simulink model "verify_AIV_WetBulbTemperature_mdl"  (R2016b)
settings: Solver=VariableStepDiscrete  StartTime=0.0  StopTime=10.0  MaxStep=0.1  RelTol=1e-3  EnableMultiTasking=on
undefined symbols (not defined in the file or in its folder): rel_hum2x
libraries: carnot x2
settings Model: Creator=drhf  LastModifiedBy=drhf
settings DataIOCC: LimitDataPoints=on  SaveFormat=Array
settings OptimizationCC: ExpressionDepthLimit=2147483647  LifeSpan=inf
settings DebuggingCC: UnderspecifiedInitializationDetection=Classic  MergeDetectMultiDrivingBlocksExec=none  SolverPrmCheckMsg=warning  StateNameClashWarn=warning  SFUnexpectedBacktrackingDiag=warning  SFNoUnconditionalDefaultTransitionDiag=warning  SFExecutionAtInitializationDiag=none
settings HardwareCC: ProdBitPerPointer=32  ProdBitPerSizeT=32  ProdBitPerPtrDiffT=32  ProdLargestAtomicFloat=None  ProdIntDivRoundTo=Undefined  ProdEndianess=Unspecified  ProdWordSize=32  ProdHWDeviceType=32-bit Generic
settings ModelReferenceCC: PropagateSignalLabelsOutOfModel=off
settings GRTTargetCC: TargetLangStandard=C89/C90 (ANSI)  GeneratePreprocessorConditionals=Disable all  CombineOutputUpdateFcns=off  GRTInterface=on
settings ConfigComp: CovMetricSettings=dw  CovHtmlReporting=on  CovSaveCumulativeToWorkspaceVar=on  CovSaveSingleToWorkspaceVar=on  CovExternalEMLEnable=off

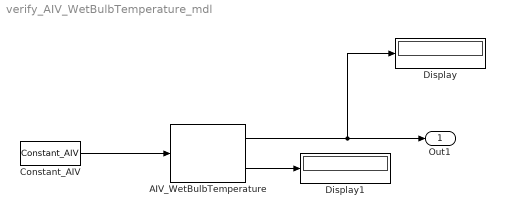
== system verify_AIV_WetBulbTemperature_mdl ==
  AIV_WetBulbTemperature : carnot/Basic/Material_Properties/AIV_WetBulbTemperature
  Constant_AIV : carnot/Source/Ventilation/Constant_AIV  Tsens=20  Tcon=20  Trad=20  mw=rel_hum2x(20,1e5,50)  mco=500/1e6  rhoair=1.2  cpair=1004  pair=100000  nair=0.5
  Display : Display
  Display1 : Display
  Out1 : Outport
  wires:
  AIV_WetBulbTemperature/1 -> Display/1, Out1/1
  AIV_WetBulbTemperature/2 -> Display1/1
  Constant_AIV/1 -> AIV_WetBulbTemperature/1
